simulink model "Simultation"  (R2023b)
settings: Solver=VariableStepAuto  StartTime=0.0  StopTime=25  RelTol=1e-3
values from neighbouring files (symbols this model uses):
  A = M1^(-1)*M2    [QUBE2_Control_System.m]
  B = M1^(-1)*M3    [QUBE2_Control_System.m]
  C = [1,0,0,0 ... (first row only)    [QUBE2_Control_System.m]
  D = 0    [QUBE2_Control_System.m]
  K = [0, 0; 0, g*l1*m1]    [QUBE2_Control_System.m]
undefined symbols (not defined in the file or in its folder): A_swingup, alpha_0, alpha_0_swingup, B_swingup, Bp_, C_swingup, D_swingup, g_, Jp_, Jr_ex_, K_lq, K_swingup, Kc_, Ke_, Lp, lp_, Lr_, mp_, mr, Ra_, theta_0, Va_0
libraries: simulink_extras x36
(part 1 of 2)
settings Model: Creator=mozar  LastModifiedBy=mozar
settings SolverCC: ZeroCrossAlgorithm=Adaptive
settings DebuggingCC: IgnoredZcDiagnostic=none

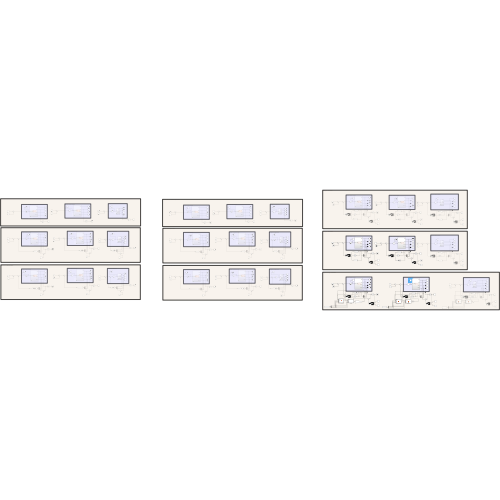
[thumbnail: Simulink's stored preview of the top-level diagram]
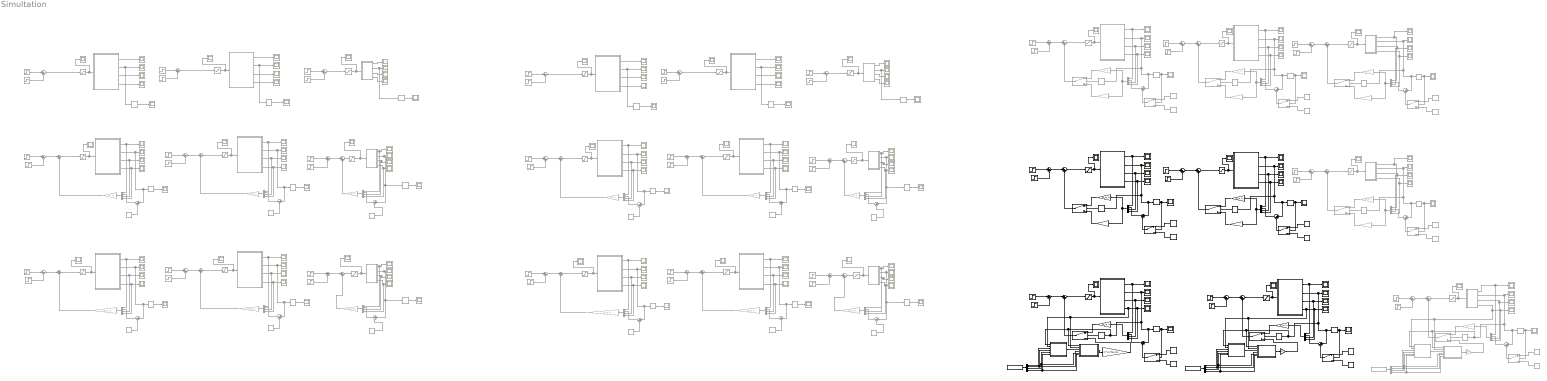
== system Simultation ==
  note: PP Swingup + PP Stabilization
  note: PP - 0 phi - 2V 0.05s Square Disturb
  note: Natual Response - 0 phi - Disturb 2V square 0.05 sec
  note: Complete Linear With Friction
  note: complete nonlinear with friction
  note: complete nonlinear no friction
  note: complete nonlinear no friction
  note: Complete Linear With Friction
  note: complete nonlinear with friction
  note: Complete Linear With Friction
  note: complete nonlinear with friction
  note: complete nonlinear no friction
  note: LQR - 0 phi - 2V 0.05s Square Disturb
  note: Complete Linear With Friction
  note: complete nonlinear with friction
  note: complete nonlinear no friction
  note: complete nonlinear no friction
  note: complete nonlinear with friction
  note: complete nonlinear no friction
  note: LQR - pi phi - 2V 0.05s Square Disturb
  note: Natual Response - pi phi - Disturb 2V square 0.05 sec
  note: complete nonlinear with friction
  note: PP - pi phi - 2V 0.05s Square Disturb
  note: Complete Linear With Friction
  note: Complete Linear With Friction
  note: complete nonlinear no friction
  note: complete nonlinear with friction
  note: Complete Linear With Friction
  note: PP Swingup + LQR Stabilization
  note: complete nonlinear no friction
  note: complete nonlinear with friction
  note: Complete Linear With Friction
  note: Energy Based Swingup + PP Stabilization
  note: complete nonlinear no friction
  note: complete nonlinear with friction
  note: complete linear with friction
  Constant{,1..12,14,17,22,31} (17 alike) : Constant  Commented=on  Value=pi
  Constant{13,18,25,28} (4 alike) : Constant  Value=pi
  Constant{15..16,19,23,32} (5 alike) : Constant  Commented=on  Value=0
  Constant{20..21,27,29} (4 alike) : Constant  Value=0
  Constant24 : Constant  Value=[Jp_ mp_ Lp g_]
  Constant26 : Constant  Value=[Jp_ mp_ Lp g_]
  Constant30 : Constant  Commented=on  Value=[Jp_ mp_ Lp g_]
  Demux1 : Demux
  Demux2 : Demux
  Demux3 : Demux  Commented=on
  Energy computation : MATLAB Function  TreatAsAtomicUnit=on
  Energy computation1 : MATLAB Function  TreatAsAtomicUnit=on
  Energy computation2 : MATLAB Function  Commented=on  TreatAsAtomicUnit=on
  Gain{1..2,6..8,12,19} (7 alike) : Gain  Commented=on  Gain=-K_lq  Multiplication=Matrix(K*u) (u vector)
  Gain{3..5,9..11,13..15,30} (10 alike) : Gain  Commented=on  Gain=-K  Multiplication=Matrix(K*u) (u vector)
  Gain{16..18,24} (4 alike) : Gain  Commented=on  Gain=-K_swingup  Multiplication=Matrix(K*u) (u vector)
  Gain{20..21,27..28} (4 alike) : Gain  Gain=-K_lq  Multiplication=Matrix(K*u) (u vector)
  Gain22 : Gain  Gain=-K_swingup  Multiplication=Matrix(K*u) (u vector)
  Gain23 : Gain  Gain=-K_swingup  Multiplication=Matrix(K*u) (u vector)
  Gain25 : Gain  Gain=mr*Lr_*Ra_/Kc_
  Gain26 : Gain  Gain=mr*Lr_*Ra_/Kc_
  Gain29 : Gain  Commented=on  Gain=mr*Lr_*Ra_/Kc_
  Mux{1..16,20} (17 alike) : Mux  Commented=on
  Mux{17..19,21} (4 alike) : Mux
  Radians to Degrees{,1..23,26,29,34..35} (28 alike) : simulink_extras/Transformations/Radians to Degrees  Commented=on
  Radians to Degrees{24..25,27..28,30..33} (8 alike) : simulink_extras/Transformations/Radians to Degrees
  Saturation{,1..6,9..15,18..20,23,26} (19 alike) : Saturate  Commented=on  UpperLimit=10  LowerLimit=-10
  Saturation{7..8,16..17} (4 alike) : Saturate  Commented=on
  Saturation{21..22,24..25} (4 alike) : Saturate  UpperLimit=10  LowerLimit=-10
  Scope{,1..113,115..126,132..135,142..143,156..161} (138 alike) : Scope  Commented=on
  Scope{114,127..131,136..141,144..155} (24 alike) : Scope
  Step{1,3,5..6,8,10,12,14,16,19..20,22,24,26,30,32..33,35,37,39,41,47,53} (23 alike) : Step  Commented=on  Before=1  After=3  SampleTime=0
  Step{2,4,7,9,11,13,15,17..18,21,23,25,27..29,31,34,36,38,40,42,48,54} (23 alike) : Step  Commented=on  Time=1.05  Before=1  After=3  SampleTime=0
  Step{43,45,49,51} (4 alike) : Step  Before=1  After=3  SampleTime=0
  Step{44,46,50,52} (4 alike) : Step  Time=1.05  Before=1  After=3  SampleTime=0
  Subsystem1 : Subsystem  Commented=on
  Subsystem10 : Subsystem  Commented=on
  Subsystem11 : Subsystem  Commented=on
  Subsystem12 : Subsystem  Commented=on
  Subsystem13 : Subsystem  Commented=on
  Subsystem14 : Subsystem
  Subsystem15 : Subsystem  Commented=on
  Subsystem16 : Subsystem
  Subsystem17 : Subsystem
  Subsystem18 : Subsystem
  Subsystem2 : Subsystem  Commented=on
  Subsystem3 : Subsystem  Commented=on
  Subsystem4 : Subsystem  Commented=on
  Subsystem5 : Subsystem  Commented=on
  Subsystem6 : Subsystem  Commented=on
  Subsystem7 : Subsystem  Commented=on
  Subsystem8 : Subsystem  Commented=on
  Subsystem9 : Subsystem  Commented=on
  Sum{1,5,7,12,16,18,22,25,29,31,38,40,43,46,49,55,67} (17 alike) : Sum  Commented=on  Inputs=|++
  Sum{2..4,6,8..11,13..15,17,19..21,23..24,26..28,30,32..37,39,41..42,44..45,47..48,50..51,56..57,68..69} (40 alike) : Sum  Commented=on  Inputs=|+-
  Sum{52,58,61,64} (4 alike) : Sum  Inputs=|++
  Sum{53..54,59..60,62..63,65..66} (8 alike) : Sum  Inputs=|+-
  Switch{,2,4,10} (4 alike) : Switch  Commented=on  Threshold=135  SaturateOnIntegerOverflow=off  InputSameDT=off
  Switch{1,3,5,11} (4 alike) : Switch  Commented=on  Criteria=u2 > Threshold  Threshold=135  SaturateOnIntegerOverflow=off  InputSameDT=off
  Switch12 : Switch  Threshold=155  SaturateOnIntegerOverflow=off  InputSameDT=off
  Switch13 : Switch  Criteria=u2 > Threshold  Threshold=155  SaturateOnIntegerOverflow=off  InputSameDT=off
  Switch{6,8,14..15} (4 alike) : Switch  Threshold=135  SaturateOnIntegerOverflow=off  InputSameDT=off
  Switch16 : Switch  Commented=on  Threshold=155  SaturateOnIntegerOverflow=off  InputSameDT=off
  Switch17 : Switch  Commented=on  Criteria=u2 > Threshold  Threshold=155  SaturateOnIntegerOverflow=off  InputSameDT=off
  Switch7 : Switch  Criteria=u2 > Threshold  Threshold=135  SaturateOnIntegerOverflow=off  InputSameDT=off
  Switch9 : Switch  Criteria=u2 > Threshold  Threshold=135  SaturateOnIntegerOverflow=off  InputSameDT=off
  linearized_model1 : Subsystem  Commented=on
  linearized_model2 : Subsystem  Commented=on
  linearized_model3 : Subsystem  Commented=on
  linearized_model4 : Subsystem  Commented=on
  linearized_model5 : Subsystem  Commented=on
  linearized_model6 : Subsystem  Commented=on
  linearized_model7 : Subsystem  Commented=on
  linearized_model8 : Subsystem  Commented=on
  linearized_model9 : Subsystem  Commented=on
  saturation : MATLAB Function  TreatAsAtomicUnit=on
  saturation1 : MATLAB Function  TreatAsAtomicUnit=on
  saturation2 : MATLAB Function  Commented=on  TreatAsAtomicUnit=on
  wires:
  linearized_model1/2(alpha) -> Radians to Degrees3/1, Scope19/1
  linearized_model1/1(theta) -> Scope18/1
  Radians to Degrees3/1 -> Scope20/1
  linearized_model1/4(alpha_d) -> Scope17/1
  linearized_model1/3(theta_d) -> Scope16/1
  Subsystem2/1(theta) -> Scope21/1
  Subsystem2/4(alpha_d) -> Scope24/1
  Sum10/1 -> Saturation2/1
  Subsystem2/2(alpha) -> Radians to Degrees4/1, Scope22/1
  Saturation2/1 -> Scope50/1, Subsystem2/1(Input_Voltage)
  Subsystem2/3(theta_d) -> Scope23/1
  Radians to Degrees4/1 -> Scope25/1
  Saturation3/1 -> Scope31/1, Subsystem3/1(Input_Voltage)
  Subsystem3/2(alpha) -> Radians to Degrees5/1, Scope27/1
  Subsystem3/3(theta_d) -> Scope28/1
  Step11/1 -> Sum9/2
  Radians to Degrees5/1 -> Scope30/1
  Step10/1 -> Sum9/1
  Subsystem3/4(alpha_d) -> Scope29/1
  Sum9/1 -> Saturation3/1
  Subsystem3/1(theta) -> Scope26/1
  Step6/1 -> Sum10/1
  Step7/1 -> Sum10/2
  Step8/1 -> Sum11/1
  Step9/1 -> Sum11/2
  Subsystem4/1(theta) -> Mux3/1, Scope32/1
  Mux3/1 -> Gain3/1
  Radians to Degrees6/1 -> Scope36/1
  Constant3/1 -> Sum14/2
  Subsystem4/4(alpha_d) -> Mux3/4, Scope35/1
  Sum12/1 -> Saturation4/1
  Subsystem4/2(alpha) -> Sum14/1, Radians to Degrees6/1, Scope33/1
  Sum14/1 -> Mux3/2
  Sum13/1 -> Sum12/1
  Saturation4/1 -> Scope/1, Subsystem4/1(Input_Voltage)
  Subsystem4/3(theta_d) -> Mux3/3, Scope34/1
  Gain3/1 -> Sum12/2
  linearized_model2/2(alpha) -> Sum15/1, Radians to Degrees7/1, Scope40/1
  Mux4/1 -> Gain4/1
  linearized_model2/1(theta) -> Mux4/1, Scope39/1
  Radians to Degrees7/1 -> Scope41/1
  Gain4/1 -> Sum16/2
  Sum17/1 -> Sum16/1
  Constant4/1 -> Sum15/2
  linearized_model2/4(alpha_d) -> Mux4/4, Scope38/1
  Sum15/1 -> Mux4/2
  linearized_model2/3(theta_d) -> Mux4/3, Scope37/1
  Subsystem5/2(alpha) -> Sum20/1, Radians to Degrees8/1, Scope43/1
  Saturation5/1 -> Scope42/1, Subsystem5/1(Input_Voltage)
  Sum19/1 -> Sum18/1
  Subsystem5/3(theta_d) -> Mux5/3, Scope44/1
  Subsystem5/4(alpha_d) -> Mux5/4, Scope45/1
  Radians to Degrees8/1 -> Scope46/1
  Subsystem5/1(theta) -> Mux5/1, Scope47/1
  Mux5/1 -> Gain5/1
  Sum18/1 -> Saturation5/1
  Constant5/1 -> Sum20/2
  Gain5/1 -> Sum18/2
  Sum20/1 -> Mux5/2
  Step12/1 -> Sum13/1
  Step13/1 -> Sum13/2
  Step14/1 -> Sum19/1
  Step15/1 -> Sum19/2
  Step16/1 -> Sum17/1
  Step17/1 -> Sum17/2
  Sum6/1 -> Sum5/1
  Sum4/1 -> Mux2/2
  Constant2/1 -> Sum4/2
  linearized_model3/4(alpha_d) -> Mux2/4, Scope7/1
  linearized_model3/3(theta_d) -> Mux2/3, Scope6/1
  Mux2/1 -> Gain2/1
  linearized_model3/1(theta) -> Mux2/1, Scope8/1
  Sum7/1 -> Saturation6/1
  Mux6/1 -> Gain6/1
  Radians to Degrees2/1 -> Scope10/1
  Sum21/1 -> Mux6/2
  Subsystem6/1(theta) -> Mux6/1, Scope15/1
  Saturation6/1 -> Scope52/1, Subsystem6/1(Input_Voltage)
  linearized_model3/2(alpha) -> Sum4/1, Radians to Degrees2/1, Scope9/1
  Subsystem6/3(theta_d) -> Mux6/3, Scope12/1
  Step5/1 -> Sum6/1
  Radians to Degrees9/1 -> Scope14/1
  Sum8/1 -> Sum7/1
  Step3/1 -> Sum8/1
  Constant6/1 -> Sum21/2
  Step1/1 -> Sum2/1
  Step2/1 -> Sum2/2
  Subsystem6/2(alpha) -> Sum21/1, Radians to Degrees9/1, Scope11/1
  Step4/1 -> Sum8/2
  Sum2/1 -> Sum1/1
  Saturation1/1 -> Scope51/1, Subsystem1/1(Input_Voltage)
  Gain6/1 -> Sum7/2
  Gain1/1 -> Sum1/2
  Gain2/1 -> Sum5/2
  Subsystem1/3(theta_d) -> Mux1/3, Scope3/1
  Constant1/1 -> Sum3/2
  Subsystem1/1(theta) -> Mux1/1, Scope1/1
  Mux1/1 -> Gain1/1
  Subsystem6/4(alpha_d) -> Mux6/4, Scope13/1
  Radians to Degrees1/1 -> Scope5/1
  Sum1/1 -> Saturation1/1
  Step18/1 -> Sum6/2
  Subsystem1/2(alpha) -> Sum3/1, Radians to Degrees1/1, Scope2/1
  Sum3/1 -> Mux1/2
  Subsystem1/4(alpha_d) -> Mux1/4, Scope4/1
  Sum16/1 -> Saturation/1
  Saturation/1 -> Scope48/1, linearized_model2/1(Va)
  Saturation7/1 -> Scope49/1, linearized_model1/1(Va)
  Sum11/1 -> Saturation7/1
  Sum5/1 -> Saturation8/1
  Saturation8/1 -> Scope53/1, linearized_model3/1(Va)
  Sum30/1 -> Sum29/1
  Sum28/1 -> Mux10/2
  Constant10/1 -> Sum28/2
  linearized_model5/4(alpha_d) -> Mux10/4, Scope86/1
  Step26/1 -> Sum30/1
  Gain10/1 -> Sum29/2
  Mux10/1 -> Gain10/1
  linearized_model5/1(theta) -> Mux10/1, Scope87/1
  linearized_model5/2(alpha) -> Sum28/1, Radians to Degrees16/1, Scope89/1
  Sum31/1 -> Saturation14/1
  Gain11/1 -> Sum31/2
  Mux11/1 -> Gain11/1
  Sum34/1 -> Mux11/2
  Subsystem11/1(theta) -> Mux11/1, Scope96/1
  Saturation14/1 -> Scope91/1, Subsystem11/1(Input_Voltage)
  Radians to Degrees17/1 -> Scope95/1
  Sum32/1 -> Sum31/1
  Subsystem11/4(alpha_d) -> Mux11/4, Scope94/1
  Subsystem11/2(alpha) -> Sum34/1, Radians to Degrees17/1, Scope92/1
  Step24/1 -> Sum32/1
  Step22/1 -> Sum26/1
  Step23/1 -> Sum26/2
  Step25/1 -> Sum32/2
  Sum26/1 -> Sum25/1
  Saturation13/1 -> Scope54/1, Subsystem10/1(Input_Voltage)
  Subsystem10/3(theta_d) -> Mux9/3, Scope82/1
  Subsystem10/1(theta) -> Mux9/1, Scope80/1
  Mux9/1 -> Gain9/1
  Sum25/1 -> Saturation13/1
  Step35/1 -> Sum24/1
  Saturation11/1 -> Scope100/1, Subsystem8/1(Input_Voltage)
  Subsystem11/3(theta_d) -> Mux11/3, Scope93/1
  Subsystem8/2(alpha) -> Radians to Degrees13/1, Scope69/1
  Subsystem8/1(theta) -> Scope68/1
  Subsystem8/3(theta_d) -> Scope70/1
  Subsystem8/4(alpha_d) -> Scope71/1
  Step36/1 -> Sum24/2
  Radians to Degrees13/1 -> Scope72/1
  Sum23/1 -> Saturation11/1
  Sum27/1 -> Mux9/2
  Step20/1 -> Sum42/1
  Step21/1 -> Sum42/2
  Constant11/1 -> Sum34/2
  Sum42/1 -> Saturation12/1
  Radians to Degrees14/1 -> Scope78/1
  Sum38/1 -> Saturation17/1
  Gain9/1 -> Sum25/2
  Saturation17/1 -> Scope103/1, linearized_model6/1(Va)
  Step27/1 -> Sum30/2
  Sum29/1 -> Saturation9/1
  Sum24/1 -> Saturation16/1
  Saturation16/1 -> Scope98/1, linearized_model4/1(Va)
  Step34/1 -> Sum23/2
  Subsystem9/1(theta) -> Scope73/1
  Subsystem9/3(theta_d) -> Scope75/1
  Constant9/1 -> Sum27/2
  Subsystem9/4(alpha_d) -> Scope76/1
  Subsystem7/4(alpha_d) -> Mux7/4, Scope88/1
  Subsystem12/4(alpha_d) -> Mux12/4, Scope59/1
  Radians to Degrees10/1 -> Scope99/1
  Mux7/1 -> Gain7/1
  Sum36/1 -> Mux7/2
  Step28/1 -> Sum39/2
  Subsystem7/3(theta_d) -> Mux7/3, Scope77/1
  Subsystem7/2(alpha) -> Sum36/1, Radians to Degrees10/1, Scope66/1
  Subsystem12/2(alpha) -> Sum35/1, Radians to Degrees18/1, Scope57/1
  Radians to Degrees15/1 -> Scope84/1
  Step29/1 -> Sum33/2
  Step31/1 -> Sum41/2
  Radians to Degrees16/1 -> Scope90/1
  Gain12/1 -> Sum40/2
  Sum33/1 -> Sum22/1
  Subsystem12/3(theta_d) -> Mux12/3, Scope58/1
  Sum41/1 -> Sum40/1
  Radians to Degrees18/1 -> Scope60/1
  Gain8/1 -> Sum38/2
  Constant12/1 -> Sum35/2
  Radians to Degrees11/1 -> Scope56/1
  Subsystem10/4(alpha_d) -> Mux9/4, Scope83/1
  Subsystem9/2(alpha) -> Radians to Degrees14/1, Scope74/1
  Sum40/1 -> Saturation15/1
  Saturation10/1 -> Scope101/1, Subsystem7/1(Input_Voltage)
  Constant7/1 -> Sum36/2
  Mux12/1 -> Gain12/1
  Subsystem12/1(theta) -> Mux12/1, Scope61/1
  Step30/1 -> Sum41/1
  Step19/1 -> Sum33/1
  linearized_model6/3(theta_d) -> Mux8/3, Scope104/1
  linearized_model6/4(alpha_d) -> Mux8/4, Scope105/1
  linearized_model6/2(alpha) -> Sum37/1, Radians to Degrees11/1, Scope107/1
  Gain7/1 -> Sum22/2
  linearized_model5/3(theta_d) -> Mux10/3, Scope85/1
  Step33/1 -> Sum23/1
  Step32/1 -> Sum39/1
  Sum39/1 -> Sum38/1
  Sum37/1 -> Mux8/2
  Subsystem7/1(theta) -> Mux7/1, Scope55/1
  Mux8/1 -> Gain8/1
  Sum22/1 -> Saturation10/1
  linearized_model6/1(theta) -> Mux8/1, Scope106/1
  Saturation12/1 -> Scope79/1, Subsystem9/1(Input_Voltage)
  linearized_model4/1(theta) -> Scope64/1
  Sum35/1 -> Mux12/2
  Saturation9/1 -> Scope97/1, linearized_model5/1(Va)
  Radians to Degrees12/1 -> Scope67/1
  linearized_model4/3(theta_d) -> Scope62/1
  Constant8/1 -> Sum37/2
  Subsystem10/2(alpha) -> Sum27/1, Radians to Degrees15/1, Scope81/1
  linearized_model4/2(alpha) -> Radians to Degrees12/1, Scope65/1
  linearized_model4/4(alpha_d) -> Scope63/1
  Saturation15/1 -> Scope102/1, Subsystem12/1(Input_Voltage)
  Step38/1 -> Sum44/2
  Radians to Degrees19/1 -> Scope113/1, Switch1/2
  Sum45/1 -> Mux15/2
  Sum43/1 -> Saturation18/1
  Saturation18/1 -> Subsystem13/1(Input_Voltage), Scope108/1
  Subsystem13/1(theta) -> Mux15/1, Scope109/1
  Subsystem13/3(theta_d) -> Mux15/3, Scope111/1
  Step37/1 -> Sum44/1
  Sum44/1 -> Sum43/1
  Subsystem13/4(alpha_d) -> Mux15/4, Scope112/1
  Subsystem13/2(alpha) -> Radians to Degrees/1, Sum45/1, Radians to Degrees19/1, Scope110/1
  Switch/1 -> Sum43/2
  Mux15/1 -> Gain16/1, Gain15/1
  Gain16/1 -> Switch/3
  Gain15/1 -> Switch/1
  Radians to Degrees/1 -> Switch/2
  Switch1/1 -> Sum45/2
  Constant/1 -> Switch1/1
  Constant15/1 -> Switch1/3
  Radians to Degrees21/1 -> Switch2/2
  Mux14/1 -> Gain17/1, Gain14/1
  Gain17/1 -> Switch2/3
  Gain14/1 -> Switch2/1
  Subsystem15/4(alpha_d) -> Mux14/4, Scope123/1
  Switch3/1 -> Sum51/2
  Subsystem15/3(theta_d) -> Mux14/3, Scope122/1
  Sum50/1 -> Sum49/1
  Subsystem15/2(alpha) -> Radians to Degrees21/1, Sum51/1, Radians to Degrees22/1, Scope121/1
  Step39/1 -> Sum50/1
  Subsystem15/1(theta) -> Mux14/1, Scope120/1
  Saturation19/1 -> Subsystem15/1(Input_Voltage), Scope119/1
  Sum49/1 -> Saturation19/1
  Radians to Degrees22/1 -> Scope124/1, Switch3/2
  Switch2/1 -> Sum49/2
  Constant14/1 -> Switch3/1
  Step40/1 -> Sum50/2
  Constant16/1 -> Switch3/3
  Sum51/1 -> Mux14/2
  linearized_model8/3(theta_d) -> Mux13/3, Scope118/1
  linearized_model8/2(alpha) -> Scope117/1, Radians to Degrees20/1, Sum48/1, Radians to Degrees23/1
  linearized_model8/1(theta) -> Scope116/1, Mux13/1
  Saturation20/1 -> linearized_model8/1(Va), Scope115/1
  Step42/1 -> Sum47/2
  Constant19/1 -> Switch5/3
  Switch4/1 -> Sum46/2
  Radians to Degrees23/1 -> Scope126/1, Switch5/2
  Sum46/1 -> Saturation20/1
  Sum47/1 -> Sum46/1
  Switch5/1 -> Sum48/2
  Step41/1 -> Sum47/1
  Sum48/1 -> Mux13/2
  Radians to Degrees20/1 -> Switch4/2
  Mux13/1 -> Gain18/1, Gain13/1
  Gain13/1 -> Switch4/1
  Gain18/1 -> Switch4/3
  linearized_model8/4(alpha_d) -> Mux13/4, Scope125/1
  Constant17/1 -> Switch5/1
  Constant22/1 -> Switch11/1
  Radians to Degrees28/1 -> Scope141/1, Switch9/2
  Sum59/1 -> Sum58/1
  Subsystem16/1(theta) -> Mux17/1, Scope137/1
  linearized_model7/1(theta) -> Scope133/1, Mux16/1
  Radians to Degrees29/1 -> Scope143/1, Switch11/2
  Constant18/1 -> Switch9/1
  Sum60/1 -> Mux17/2
  Constant20/1 -> Switch7/3
  Step44/1 -> Sum53/2
  Step46/1 -> Sum59/2
  Switch8/1 -> Sum58/2
  Step43/1 -> Sum53/1
  Sum52/1 -> Saturation21/1
  Radians to Degrees25/1 -> Scope131/1, Switch7/2
  Subsystem16/4(alpha_d) -> Mux17/4, Scope140/1
  Switch9/1 -> Sum60/2
  Gain20/1 -> Switch8/1
  Constant13/1 -> Switch7/1
  Gain22/1 -> Switch6/3
  Switch6/1 -> Sum52/2
  Sum58/1 -> Saturation22/1
  Mux16/1 -> Gain24/1, Gain19/1
  Step48/1 -> Sum56/2
  linearized_model7/2(alpha) -> Scope134/1, Radians to Degrees26/1, Sum57/1, Radians to Degrees29/1
  Radians to Degrees27/1 -> Switch8/2
  Gain19/1 -> Switch10/1
  Subsystem16/3(theta_d) -> Mux17/3, Scope139/1
  Sum53/1 -> Sum52/1
  Mux17/1 -> Gain23/1, Gain20/1
  Radians to Degrees26/1 -> Switch10/2
  Constant21/1 -> Switch9/3
  Subsystem16/2(alpha) -> Radians to Degrees27/1, Sum60/1, Radians to Degrees28/1, Scope138/1
  Sum57/1 -> Mux16/2
  linearized_model7/3(theta_d) -> Mux16/3, Scope135/1
  Step47/1 -> Sum56/1
  Saturation21/1 -> Subsystem14/1(Input_Voltage), Scope114/1
  Saturation22/1 -> Subsystem16/1(Input_Voltage), Scope136/1
  Gain21/1 -> Switch6/1
  Constant23/1 -> Switch11/3
  Switch10/1 -> Sum55/2
  Switch7/1 -> Sum54/2
  Sum56/1 -> Sum55/1
  Sum55/1 -> Saturation23/1
  Sum54/1 -> Mux18/2
  Saturation23/1 -> linearized_model7/1(Va), Scope132/1
  Switch11/1 -> Sum57/2
  Radians to Degrees24/1 -> Switch6/2
  Step45/1 -> Sum59/1
  Gain24/1 -> Switch10/3
  linearized_model7/4(alpha_d) -> Mux16/4, Scope142/1
  Subsystem14/1(theta) -> Mux18/1, Scope127/1
  Subsystem14/4(alpha_d) -> Mux18/4, Scope130/1
  Gain23/1 -> Switch8/3
  Subsystem14/2(alpha) -> Radians to Degrees24/1, Sum54/1, Radians to Degrees25/1, Scope128/1
  Subsystem14/3(theta_d) -> Mux18/3, Scope129/1
  Mux18/1 -> Gain22/1, Gain21/1
  Demux2/4 -> Energy computation/6(g0), saturation/6(g0)
  saturation/1(u) -> Gain25/1
  Constant24/1 -> Demux2/1
  Demux2/1 -> Energy computation/3(Ip)
  Energy computation/1(E) -> saturation/3(E)
  Demux2/2 -> saturation/4(mp), Energy computation/4(mp)
  Demux2/3 -> saturation/5(Lp), Energy computation/5(Lp)
  Radians to Degrees31/1 -> Scope149/1, Switch15/2
  Constant27/1 -> Switch15/3
  Step50/1 -> Sum62/2
  Subsystem17/2(alpha) -> saturation/1(phi), Energy computation/1(phi), Radians to Degrees30/1, Sum63/1, Radians to Degrees31/1, Scope146/1
  Subsystem17/3(theta_d) -> Mux21/3, Scope147/1
  Mux21/1 -> Gain28/1
  Subsystem17/1(theta) -> Mux21/1, Scope145/1
  Radians to Degrees30/1 -> Switch14/2
  Sum63/1 -> Mux21/2
  Step49/1 -> Sum62/1
  Sum61/1 -> Saturation24/1
  Saturation24/1 -> Subsystem17/1(Input_Voltage), Scope144/1
  Subsystem17/4(alpha_d) -> saturation/2(phi_dot), Energy computation/2(phi_dot), Mux21/4, Scope148/1
  Sum62/1 -> Sum61/1
  Switch14/1 -> Sum61/2
  Constant25/1 -> Switch15/1
  Switch15/1 -> Sum63/2
  Gain28/1 -> Switch14/1
  Gain25/1 -> Switch14/3
  saturation1/1(u) -> Gain26/1
  Gain27/1 -> Switch12/1
  Constant26/1 -> Demux1/1
  Sum65/1 -> Sum64/1
  Saturation25/1 -> Subsystem18/1(Input_Voltage), Scope150/1
  Switch13/1 -> Sum66/2
  Constant28/1 -> Switch13/1
  Demux1/3 -> saturation1/5(Lp), Energy computation1/5(Lp)
  Demux1/2 -> saturation1/4(mp), Energy computation1/4(mp)
  Demux1/4 -> Energy computation1/6(g0), saturation1/6(g0)
  Demux1/1 -> Energy computation1/3(Ip)
  Switch12/1 -> Sum64/2
  Sum66/1 -> Mux19/2
  Subsystem18/4(alpha_d) -> Mux19/4, Scope154/1, saturation1/2(phi_dot), Energy computation1/2(phi_dot)
  Radians to Degrees33/1 -> Scope155/1, Switch13/2
  Mux19/1 -> Gain27/1
  Gain26/1 -> Switch12/3
  Subsystem18/1(theta) -> Mux19/1, Scope151/1
  Subsystem18/2(alpha) -> saturation1/1(phi), Energy computation1/1(phi), Radians to Degrees32/1, Sum66/1, Radians to Degrees33/1, Scope152/1
  Sum64/1 -> Saturation25/1
  Constant29/1 -> Switch13/3
  Subsystem18/3(theta_d) -> Mux19/3, Scope153/1
  Energy computation1/1(E) -> saturation1/3(E)
  Radians to Degrees32/1 -> Switch12/2
  Step51/1 -> Sum65/1
  Step52/1 -> Sum65/2
  saturation2/1(u) -> Gain29/1
  Gain30/1 -> Switch16/1
  Constant30/1 -> Demux3/1
  Sum68/1 -> Sum67/1
  Saturation26/1 -> linearized_model9/1(Va), Scope156/1
  Switch17/1 -> Sum69/2
  Constant31/1 -> Switch17/1
  Demux3/3 -> saturation2/5(Lp), Energy computation2/5(Lp)
  Demux3/2 -> saturation2/4(mp), Energy computation2/4(mp)
  Demux3/4 -> Energy computation2/6(g0), saturation2/6(g0)
  Demux3/1 -> Energy computation2/3(Ip)
  Switch16/1 -> Sum67/2
  Sum69/1 -> Mux20/2
  linearized_model9/4(alpha_d) -> saturation2/2(phi_dot), Energy computation2/2(phi_dot), Mux20/4, Scope160/1
  Radians to Degrees35/1 -> Scope161/1, Switch17/2
  Mux20/1 -> Gain30/1
  Gain29/1 -> Switch16/3
  linearized_model9/1(theta) -> Mux20/1, Scope157/1
  linearized_model9/2(alpha) -> Scope158/1, saturation2/1(phi), Energy computation2/1(phi), Radians to Degrees34/1, Sum69/1, Radians to Degrees35/1
  Sum67/1 -> Saturation26/1
  Constant32/1 -> Switch17/3
  linearized_model9/3(theta_d) -> Mux20/3, Scope159/1
  Energy computation2/1(E) -> saturation2/3(E)
  Radians to Degrees34/1 -> Switch16/2
  Step53/1 -> Sum68/1
  Step54/1 -> Sum68/2

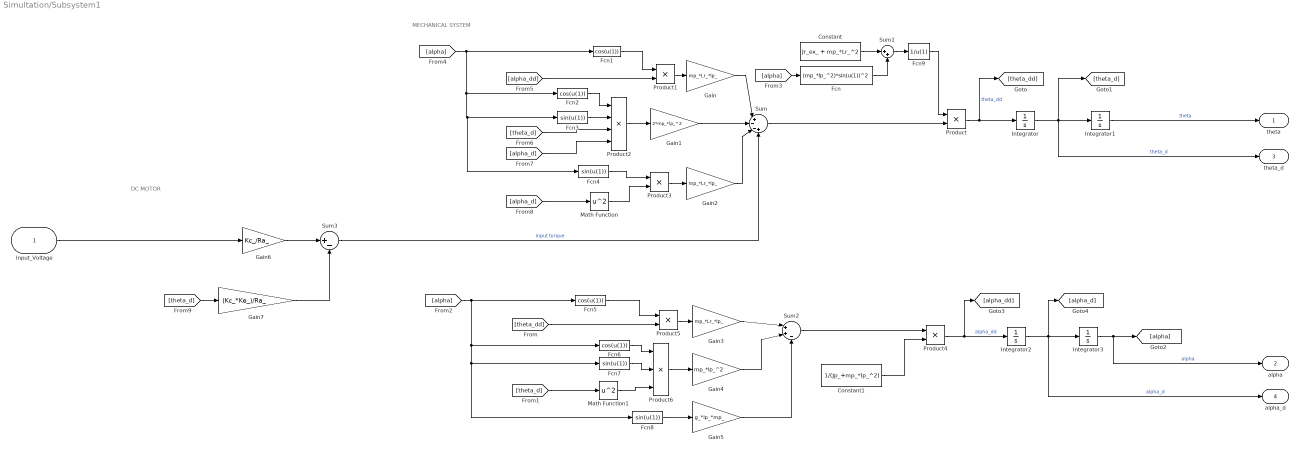
== system Simultation/Subsystem1 ==
  note: DC MOTOR
  note: MECHANICAL SYSTEM
  Input_Voltage : Inport
  Constant : Constant  Value=Jr_ex_ + mp_*Lr_^2
  Constant1 : Constant  Value=1/(Jp_+mp_*lp_^2)
  Fcn : Fcn  Expr=(mp_*lp_^2)*sin(u(1))^2
  Fcn{1..2,5..6} (4 alike) : Fcn  Expr=cos(u(1))
  Fcn{3..4,7..8} (4 alike) : Fcn  Expr=sin(u(1))
  Fcn9 : Fcn  Expr=1/u(1)
  Gain : Gain  Gain=mp_*Lr_*lp_
  Gain1 : Gain  Gain=2*mp_*lp_^2
  Gain2 : Gain  Gain=mp_*Lr_*lp_
  Gain3 : Gain  Gain=mp_*Lr_*lp_
  Gain4 : Gain  Gain=mp_*lp_^2
  Gain5 : Gain  Gain=g_*lp_*mp_
  Gain6 : Gain  Gain=Kc_/Ra_
  Gain7 : Gain  Gain=(Kc_*Ke_)/Ra_
  Integrator{,1..3} (4 alike) : Integrator
  Math Function : Math  Operator=square
  Math Function1 : Math  Operator=square
  Product{,1,3..5} (5 alike) : Product
  Product2 : Product  Inputs=4
  Product6 : Product  Inputs=3
  Sum : Sum  Inputs=|+--+
  Sum1 : Sum  Inputs=|++
  Sum2 : Sum  Inputs=|++-
  Sum3 : Sum  Inputs=|+-
  theta : Outport
  alpha : Outport  Port=2
  theta_d : Outport  Port=3
  alpha_d : Outport  Port=4
  wires:
  Integrator2/1 -> alpha_d/1, Integrator3/1, [alpha_d]  "alpha_d"
  Fcn6/1 -> Product6/1
  Product4/1 -> [alpha_dd], Integrator2/1  "alpha_dd"
  Fcn4/1 -> Product3/1
  Integrator/1 -> theta_d/1, [theta_d], Integrator1/1  "theta_d"
  Gain1/1 -> Sum/2
  Gain6/1 -> Sum3/1
  Fcn3/1 -> Product2/2
  Fcn1/1 -> Product1/1
  Integrator1/1 -> theta/1  "theta"
  Fcn8/1 -> Gain5/1
  Fcn7/1 -> Product6/2
  Gain5/1 -> Sum2/3
  Sum1/1 -> Fcn9/1
  Fcn/1 -> Sum1/2
  Product1/1 -> Gain/1
  Fcn9/1 -> Product/1
  Product3/1 -> Gain2/1
  Sum/1 -> Product/2
  [alpha_d] -> Math Function/1
  [theta_dd] -> Product5/2
  [theta_d] -> Gain7/1
  Product5/1 -> Gain3/1
  Integrator3/1 -> alpha/1, [alpha]  "alpha"
  Fcn5/1 -> Product5/1
  Product6/1 -> Gain4/1
  Sum2/1 -> Product4/1
  Math Function1/1 -> Product6/3
  Math Function/1 -> Product3/2
  Product/1 -> Integrator/1, [theta_dd]  "theta_dd"
  Gain4/1 -> Sum2/2
  Input_Voltage/1 -> Gain6/1
  Constant/1 -> Sum1/1
  [alpha] -> Fcn8/1, Fcn7/1, Fcn6/1, Fcn5/1
  Constant1/1 -> Product4/2
  Product2/1 -> Gain1/1
  [alpha] -> Fcn4/1, Fcn3/1, Fcn2/1, Fcn1/1
  [alpha_d] -> Product2/4
  [alpha_dd] -> Product1/2
  [alpha] -> Fcn/1
  Fcn2/1 -> Product2/1
  Sum3/1 -> Sum/4  "input torque"
  Gain2/1 -> Sum/3
  Gain/1 -> Sum/1
  Gain3/1 -> Sum2/1
  [theta_d] -> Math Function1/1
  Gain7/1 -> Sum3/2
  [theta_d] -> Product2/3

== system Simultation/Subsystem10 ==
  note: DC MOTOR
  note: MECHANICAL SYSTEM
  Input_Voltage : Inport
  Constant : Constant  Value=Jr_ex_ + mp_*Lr_^2
  Constant1 : Constant  Value=1/(Jp_+mp_*lp_^2)
  Fcn : Fcn  Expr=(mp_*lp_^2)*sin(u(1))^2
  Fcn{1..2,5..6} (4 alike) : Fcn  Expr=cos(u(1))
  Fcn{3..4,7..8} (4 alike) : Fcn  Expr=sin(u(1))
  Fcn9 : Fcn  Expr=1/u(1)
  Gain : Gain  Gain=mp_*Lr_*lp_
  Gain1 : Gain  Gain=2*mp_*lp_^2
  Gain2 : Gain  Gain=mp_*Lr_*lp_
  Gain3 : Gain  Gain=mp_*Lr_*lp_
  Gain4 : Gain  Gain=mp_*lp_^2
  Gain5 : Gain  Gain=g_*lp_*mp_
  Gain6 : Gain  Gain=Kc_/Ra_
  Gain7 : Gain  Gain=(Kc_*Ke_)/Ra_
  Integrator : Integrator
  Integrator1 : Integrator
  Integrator2 : Integrator
  Integrator3 : Integrator  InitialCondition=pi
  Math Function : Math  Operator=square
  Math Function1 : Math  Operator=square
  Product{,1,3..5} (5 alike) : Product
  Product2 : Product  Inputs=4
  Product6 : Product  Inputs=3
  Sum : Sum  Inputs=|+--+
  Sum1 : Sum  Inputs=|++
  Sum2 : Sum  Inputs=|++-
  Sum3 : Sum  Inputs=|+-
  theta : Outport
  alpha : Outport  Port=2
  theta_d : Outport  Port=3
  alpha_d : Outport  Port=4
  wires:
  Integrator2/1 -> alpha_d/1, Integrator3/1, [alpha_d]  "alpha_d"
  Fcn6/1 -> Product6/1
  Product4/1 -> [alpha_dd], Integrator2/1  "alpha_dd"
  Fcn4/1 -> Product3/1
  Integrator/1 -> theta_d/1, [theta_d], Integrator1/1  "theta_d"
  Gain1/1 -> Sum/2
  Gain6/1 -> Sum3/1
  Fcn3/1 -> Product2/2
  Fcn1/1 -> Product1/1
  Integrator1/1 -> theta/1  "theta"
  Fcn8/1 -> Gain5/1
  Fcn7/1 -> Product6/2
  Gain5/1 -> Sum2/3
  Sum1/1 -> Fcn9/1
  Fcn/1 -> Sum1/2
  Product1/1 -> Gain/1
  Fcn9/1 -> Product/1
  Product3/1 -> Gain2/1
  Sum/1 -> Product/2
  [alpha_d] -> Math Function/1
  [theta_dd] -> Product5/2
  [theta_d] -> Gain7/1
  Product5/1 -> Gain3/1
  Integrator3/1 -> alpha/1, [alpha]  "alpha"
  Fcn5/1 -> Product5/1
  Product6/1 -> Gain4/1
  Sum2/1 -> Product4/1
  Math Function1/1 -> Product6/3
  Math Function/1 -> Product3/2
  Product/1 -> Integrator/1, [theta_dd]  "theta_dd"
  Gain4/1 -> Sum2/2
  Input_Voltage/1 -> Gain6/1
  Constant/1 -> Sum1/1
  [alpha] -> Fcn8/1, Fcn7/1, Fcn6/1, Fcn5/1
  Constant1/1 -> Product4/2
  Product2/1 -> Gain1/1
  [alpha] -> Fcn4/1, Fcn3/1, Fcn2/1, Fcn1/1
  [alpha_d] -> Product2/4
  [alpha_dd] -> Product1/2
  [alpha] -> Fcn/1
  Fcn2/1 -> Product2/1
  Sum3/1 -> Sum/4  "input torque"
  Gain2/1 -> Sum/3
  Gain/1 -> Sum/1
  Gain3/1 -> Sum2/1
  [theta_d] -> Math Function1/1
  Gain7/1 -> Sum3/2
  [theta_d] -> Product2/3

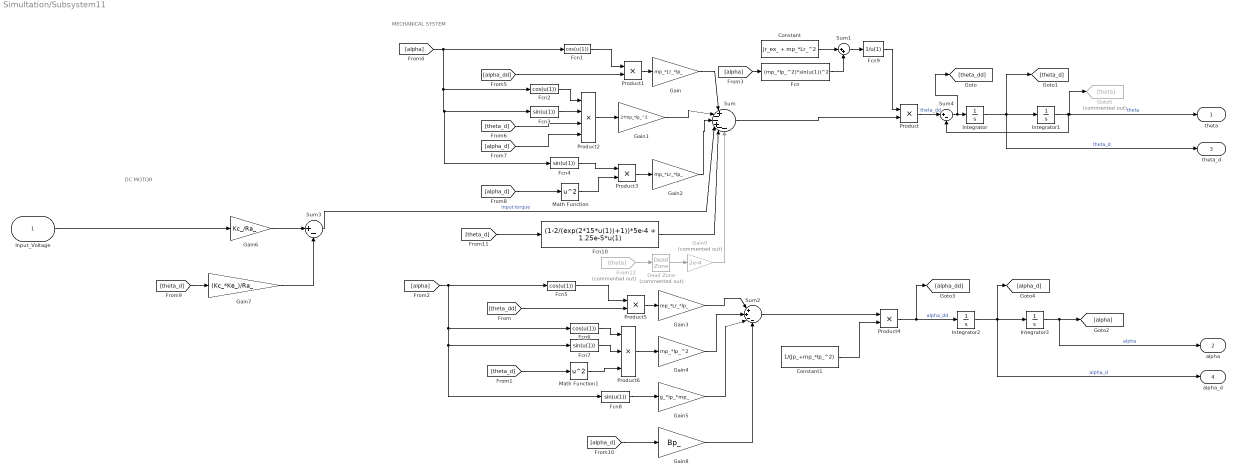
== system Simultation/Subsystem11 ==
  note: MECHANICAL SYSTEM
  note: DC MOTOR
  Input_Voltage : Inport
  Constant : Constant  Value=Jr_ex_ + mp_*Lr_^2
  Constant1 : Constant  Value=1/(Jp_+mp_*lp_^2)
  Dead Zone : DeadZone  Commented=on  LowerValue=0  UpperValue=0  ZeroCross=off
  Fcn : Fcn  Expr=(mp_*lp_^2)*sin(u(1))^2
  Fcn{1..2,5..6} (4 alike) : Fcn  Expr=cos(u(1))
  Fcn10 : Fcn  Expr=(1-2/(exp(2*15*u(1))+1))*5e-4 + 1.25e-5*u(1)
  Fcn{3..4,7..8} (4 alike) : Fcn  Expr=sin(u(1))
  Fcn9 : Fcn  Expr=1/u(1)
  From12 : From  Commented=on  GotoTag=theta
  Gain : Gain  Gain=mp_*Lr_*lp_
  Gain1 : Gain  Gain=2*mp_*lp_^2
  Gain2 : Gain  Gain=mp_*Lr_*lp_
  Gain3 : Gain  Gain=mp_*Lr_*lp_
  Gain4 : Gain  Gain=mp_*lp_^2
  Gain5 : Gain  Gain=g_*lp_*mp_
  Gain6 : Gain  Gain=Kc_/Ra_
  Gain7 : Gain  Gain=(Kc_*Ke_)/Ra_
  Gain8 : Gain  Gain=Bp_
  Gain9 : Gain  Commented=on  Gain=2e-4
  Goto5 : Goto  Commented=on  GotoTag=theta
  Integrator : Integrator
  Integrator1 : Integrator
  Integrator2 : Integrator
  Integrator3 : Integrator  InitialCondition=pi
  Math Function : Math  Operator=square
  Math Function1 : Math  Operator=square
  Product{,1,3..5} (5 alike) : Product
  Product2 : Product  Inputs=4
  Product6 : Product  Inputs=3
  Sum : Sum  Inputs=|+--+--
  Sum1 : Sum  Inputs=|++
  Sum2 : Sum  Inputs=|++--
  Sum3 : Sum  Inputs=|+-
  Sum4 : Sum  Inputs=|+-
  theta : Outport
  alpha : Outport  Port=2
  theta_d : Outport  Port=3
  alpha_d : Outport  Port=4
  wires:
  [theta_d] -> Product2/3
  Gain7/1 -> Sum3/2
  [theta_d] -> Math Function1/1
  Gain3/1 -> Sum2/1
  Gain/1 -> Sum/1
  Gain2/1 -> Sum/3
  Sum3/1 -> Sum/4  "input torque"
  Fcn2/1 -> Product2/1
  [alpha] -> Fcn/1
  [alpha_dd] -> Product1/2
  [alpha_d] -> Product2/4
  [alpha] -> Fcn1/1, Fcn2/1, Fcn3/1, Fcn4/1
  Product2/1 -> Gain1/1
  Constant1/1 -> Product4/2
  [alpha] -> Fcn5/1, Fcn6/1, Fcn7/1, Fcn8/1
  Constant/1 -> Sum1/1
  Input_Voltage/1 -> Gain6/1
  Gain4/1 -> Sum2/2
  Product/1 -> Sum4/1  "theta_dd"
  Math Function/1 -> Product3/2
  Math Function1/1 -> Product6/3
  Sum2/1 -> Product4/1
  Product6/1 -> Gain4/1
  Fcn5/1 -> Product5/1
  Integrator3/1 -> alpha/1, [alpha]  "alpha"
  Product5/1 -> Gain3/1
  [theta_d] -> Gain7/1
  [theta_dd] -> Product5/2
  [alpha_d] -> Math Function/1
  Sum/1 -> Product/2
  Product3/1 -> Gain2/1
  Fcn9/1 -> Product/1
  Product1/1 -> Gain/1
  Fcn/1 -> Sum1/2
  Sum1/1 -> Fcn9/1
  Gain5/1 -> Sum2/3
  Fcn7/1 -> Product6/2
  Fcn8/1 -> Gain5/1
  Fcn1/1 -> Product1/1
  Fcn3/1 -> Product2/2
  Gain6/1 -> Sum3/1
  Gain1/1 -> Sum/2
  Integrator/1 -> Integrator1/1, [theta_d], theta_d/1  "theta_d"
  Fcn4/1 -> Product3/1
  Product4/1 -> Integrator2/1, [alpha_dd]  "alpha_dd"
  Fcn6/1 -> Product6/1
  Integrator2/1 -> [alpha_d], Integrator3/1, alpha_d/1  "alpha_d"
  [alpha_d] -> Gain8/1
  Gain8/1 -> Sum2/4
  Integrator1/1 -> theta/1, Goto5/1, Sum4/2  "theta"
  Dead Zone/1 -> Gain9/1
  [theta_d] -> Fcn10/1
  Fcn10/1 -> Sum/5
  Gain9/1 -> Sum/6
  From12/1 -> Dead Zone/1
  Sum4/1 -> [theta_dd], Integrator/1

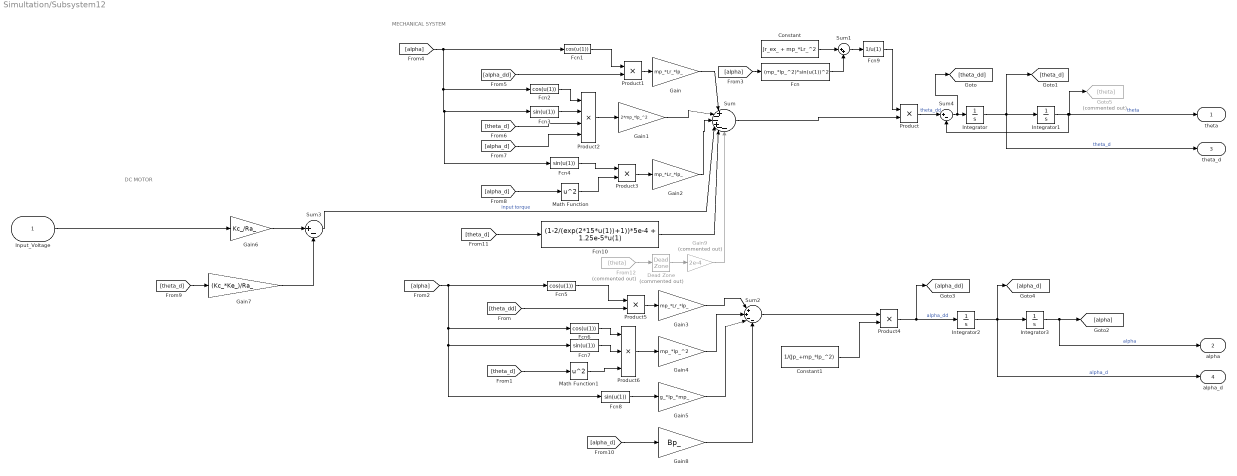
== system Simultation/Subsystem12 ==
  note: MECHANICAL SYSTEM
  note: DC MOTOR
  Input_Voltage : Inport
  Constant : Constant  Value=Jr_ex_ + mp_*Lr_^2
  Constant1 : Constant  Value=1/(Jp_+mp_*lp_^2)
  Dead Zone : DeadZone  Commented=on  LowerValue=0  UpperValue=0  ZeroCross=off
  Fcn : Fcn  Expr=(mp_*lp_^2)*sin(u(1))^2
  Fcn{1..2,5..6} (4 alike) : Fcn  Expr=cos(u(1))
  Fcn10 : Fcn  Expr=(1-2/(exp(2*15*u(1))+1))*5e-4 + 1.25e-5*u(1)
  Fcn{3..4,7..8} (4 alike) : Fcn  Expr=sin(u(1))
  Fcn9 : Fcn  Expr=1/u(1)
  From12 : From  Commented=on  GotoTag=theta
  Gain : Gain  Gain=mp_*Lr_*lp_
  Gain1 : Gain  Gain=2*mp_*lp_^2
  Gain2 : Gain  Gain=mp_*Lr_*lp_
  Gain3 : Gain  Gain=mp_*Lr_*lp_
  Gain4 : Gain  Gain=mp_*lp_^2
  Gain5 : Gain  Gain=g_*lp_*mp_
  Gain6 : Gain  Gain=Kc_/Ra_
  Gain7 : Gain  Gain=(Kc_*Ke_)/Ra_
  Gain8 : Gain  Gain=Bp_
  Gain9 : Gain  Commented=on  Gain=2e-4
  Goto5 : Goto  Commented=on  GotoTag=theta
  Integrator : Integrator
  Integrator1 : Integrator
  Integrator2 : Integrator
  Integrator3 : Integrator  InitialCondition=pi
  Math Function : Math  Operator=square
  Math Function1 : Math  Operator=square
  Product{,1,3..5} (5 alike) : Product
  Product2 : Product  Inputs=4
  Product6 : Product  Inputs=3
  Sum : Sum  Inputs=|+--+--
  Sum1 : Sum  Inputs=|++
  Sum2 : Sum  Inputs=|++--
  Sum3 : Sum  Inputs=|+-
  Sum4 : Sum  Inputs=|+-
  theta : Outport
  alpha : Outport  Port=2
  theta_d : Outport  Port=3
  alpha_d : Outport  Port=4
  wires:
  [theta_d] -> Product2/3
  Gain7/1 -> Sum3/2
  [theta_d] -> Math Function1/1
  Gain3/1 -> Sum2/1
  Gain/1 -> Sum/1
  Gain2/1 -> Sum/3
  Sum3/1 -> Sum/4  "input torque"
  Fcn2/1 -> Product2/1
  [alpha] -> Fcn/1
  [alpha_dd] -> Product1/2
  [alpha_d] -> Product2/4
  [alpha] -> Fcn1/1, Fcn2/1, Fcn3/1, Fcn4/1
  Product2/1 -> Gain1/1
  Constant1/1 -> Product4/2
  [alpha] -> Fcn5/1, Fcn6/1, Fcn7/1, Fcn8/1
  Constant/1 -> Sum1/1
  Input_Voltage/1 -> Gain6/1
  Gain4/1 -> Sum2/2
  Product/1 -> Sum4/1  "theta_dd"
  Math Function/1 -> Product3/2
  Math Function1/1 -> Product6/3
  Sum2/1 -> Product4/1
  Product6/1 -> Gain4/1
  Fcn5/1 -> Product5/1
  Integrator3/1 -> alpha/1, [alpha]  "alpha"
  Product5/1 -> Gain3/1
  [theta_d] -> Gain7/1
  [theta_dd] -> Product5/2
  [alpha_d] -> Math Function/1
  Sum/1 -> Product/2
  Product3/1 -> Gain2/1
  Fcn9/1 -> Product/1
  Product1/1 -> Gain/1
  Fcn/1 -> Sum1/2
  Sum1/1 -> Fcn9/1
  Gain5/1 -> Sum2/3
  Fcn7/1 -> Product6/2
  Fcn8/1 -> Gain5/1
  Fcn1/1 -> Product1/1
  Fcn3/1 -> Product2/2
  Gain6/1 -> Sum3/1
  Gain1/1 -> Sum/2
  Integrator/1 -> Integrator1/1, [theta_d], theta_d/1  "theta_d"
  Fcn4/1 -> Product3/1
  Product4/1 -> Integrator2/1, [alpha_dd]  "alpha_dd"
  Fcn6/1 -> Product6/1
  Integrator2/1 -> [alpha_d], Integrator3/1, alpha_d/1  "alpha_d"
  [alpha_d] -> Gain8/1
  Gain8/1 -> Sum2/4
  Integrator1/1 -> theta/1, Goto5/1, Sum4/2  "theta"
  Dead Zone/1 -> Gain9/1
  [theta_d] -> Fcn10/1
  Fcn10/1 -> Sum/5
  Gain9/1 -> Sum/6
  From12/1 -> Dead Zone/1
  Sum4/1 -> [theta_dd], Integrator/1

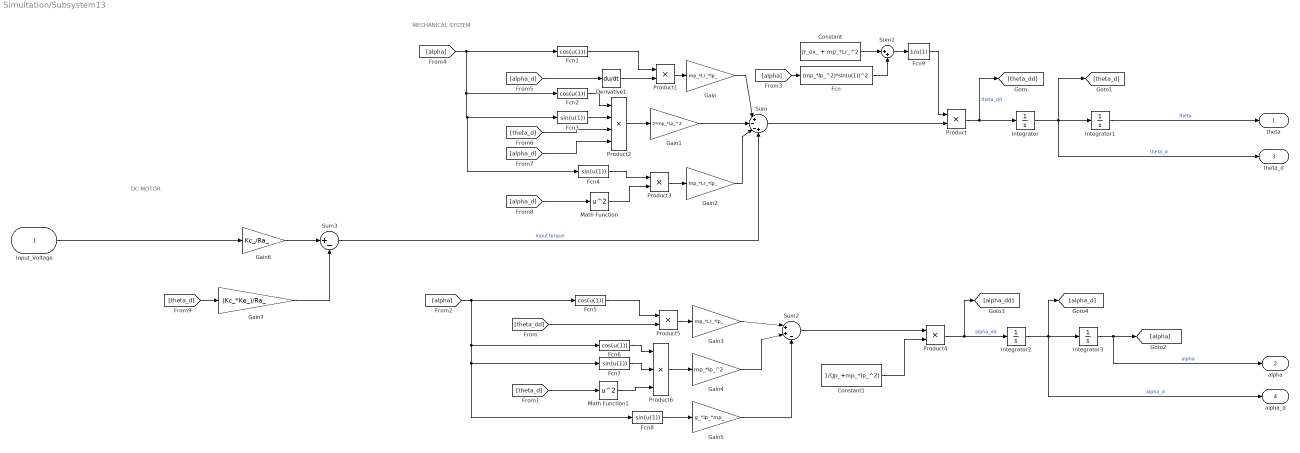
== system Simultation/Subsystem13 ==
  note: DC MOTOR
  note: MECHANICAL SYSTEM
  Input_Voltage : Inport
  Constant : Constant  Value=Jr_ex_ + mp_*Lr_^2
  Constant1 : Constant  Value=1/(Jp_+mp_*lp_^2)
  Derivative1 : Derivative
  Fcn : Fcn  Expr=(mp_*lp_^2)*sin(u(1))^2
  Fcn{1..2,5..6} (4 alike) : Fcn  Expr=cos(u(1))
  Fcn{3..4,7..8} (4 alike) : Fcn  Expr=sin(u(1))
  Fcn9 : Fcn  Expr=1/u(1)
  Gain : Gain  Gain=mp_*Lr_*lp_
  Gain1 : Gain  Gain=2*mp_*lp_^2
  Gain2 : Gain  Gain=mp_*Lr_*lp_
  Gain3 : Gain  Gain=mp_*Lr_*lp_
  Gain4 : Gain  Gain=mp_*lp_^2
  Gain5 : Gain  Gain=g_*lp_*mp_
  Gain6 : Gain  Gain=Kc_/Ra_
  Gain7 : Gain  Gain=(Kc_*Ke_)/Ra_
  Integrator{,1..3} (4 alike) : Integrator
  Math Function : Math  Operator=square
  Math Function1 : Math  Operator=square
  Product{,1,3..5} (5 alike) : Product
  Product2 : Product  Inputs=4
  Product6 : Product  Inputs=3
  Sum : Sum  Inputs=|+--+
  Sum1 : Sum  Inputs=|++
  Sum2 : Sum  Inputs=|++-
  Sum3 : Sum  Inputs=|+-
  theta : Outport
  alpha : Outport  Port=2
  theta_d : Outport  Port=3
  alpha_d : Outport  Port=4
  wires:
  Integrator2/1 -> alpha_d/1, Integrator3/1, [alpha_d]  "alpha_d"
  Fcn6/1 -> Product6/1
  Product4/1 -> [alpha_dd], Integrator2/1  "alpha_dd"
  Fcn4/1 -> Product3/1
  Integrator/1 -> theta_d/1, [theta_d], Integrator1/1  "theta_d"
  Gain6/1 -> Sum3/1
  Fcn3/1 -> Product2/2
  Fcn1/1 -> Product1/1
  Integrator1/1 -> theta/1  "theta"
  Fcn8/1 -> Gain5/1
  Fcn7/1 -> Product6/2
  Gain5/1 -> Sum2/3
  Sum1/1 -> Fcn9/1
  Fcn/1 -> Sum1/2
  Product1/1 -> Gain/1
  Fcn9/1 -> Product/1
  Product3/1 -> Gain2/1
  Sum/1 -> Product/2
  [alpha_d] -> Math Function/1
  [theta_dd] -> Product5/2
  [theta_d] -> Gain7/1
  Product5/1 -> Gain3/1
  Integrator3/1 -> alpha/1, [alpha]  "alpha"
  Fcn5/1 -> Product5/1
  Product6/1 -> Gain4/1
  Sum2/1 -> Product4/1
  Math Function1/1 -> Product6/3
  Math Function/1 -> Product3/2
  Product/1 -> Integrator/1, [theta_dd]  "theta_dd"
  Gain4/1 -> Sum2/2
  Input_Voltage/1 -> Gain6/1
  Constant/1 -> Sum1/1
  [alpha] -> Fcn8/1, Fcn7/1, Fcn6/1, Fcn5/1
  Constant1/1 -> Product4/2
  Product2/1 -> Gain1/1
  [alpha] -> Fcn4/1, Fcn3/1, Fcn2/1, Fcn1/1
  [alpha_d] -> Product2/4
  [alpha] -> Fcn/1
  Fcn2/1 -> Product2/1
  Sum3/1 -> Sum/4  "input torque"
  Gain2/1 -> Sum/3
  Gain3/1 -> Sum2/1
  [theta_d] -> Math Function1/1
  Gain7/1 -> Sum3/2
  [theta_d] -> Product2/3
  Gain1/1 -> Sum/2
  Gain/1 -> Sum/1
  [alpha_d] -> Derivative1/1
  Derivative1/1 -> Product1/2

== system Simultation/Subsystem14 ==
  note: DC MOTOR
  note: MECHANICAL SYSTEM
  Input_Voltage : Inport
  Constant : Constant  Value=Jr_ex_ + mp_*Lr_^2
  Constant1 : Constant  Value=1/(Jp_+mp_*lp_^2)
  Derivative1 : Derivative
  Fcn : Fcn  Expr=(mp_*lp_^2)*sin(u(1))^2
  Fcn{1..2,5..6} (4 alike) : Fcn  Expr=cos(u(1))
  Fcn{3..4,7..8} (4 alike) : Fcn  Expr=sin(u(1))
  Fcn9 : Fcn  Expr=1/u(1)
  Gain : Gain  Gain=mp_*Lr_*lp_
  Gain1 : Gain  Gain=2*mp_*lp_^2
  Gain2 : Gain  Gain=mp_*Lr_*lp_
  Gain3 : Gain  Gain=mp_*Lr_*lp_
  Gain4 : Gain  Gain=mp_*lp_^2
  Gain5 : Gain  Gain=g_*lp_*mp_
  Gain6 : Gain  Gain=Kc_/Ra_
  Gain7 : Gain  Gain=(Kc_*Ke_)/Ra_
  Integrator{,1..3} (4 alike) : Integrator
  Math Function : Math  Operator=square
  Math Function1 : Math  Operator=square
  Product{,1,3..5} (5 alike) : Product
  Product2 : Product  Inputs=4
  Product6 : Product  Inputs=3
  Sum : Sum  Inputs=|+--+
  Sum1 : Sum  Inputs=|++
  Sum2 : Sum  Inputs=|++-
  Sum3 : Sum  Inputs=|+-
  theta : Outport
  alpha : Outport  Port=2
  theta_d : Outport  Port=3
  alpha_d : Outport  Port=4
  wires:
  Integrator2/1 -> alpha_d/1, Integrator3/1, [alpha_d]  "alpha_d"
  Fcn6/1 -> Product6/1
  Product4/1 -> Integrator2/1  "alpha_dd"
  Fcn4/1 -> Product3/1
  Integrator/1 -> theta_d/1, [theta_d], Integrator1/1  "theta_d"
  Gain6/1 -> Sum3/1
  Fcn3/1 -> Product2/2
  Fcn1/1 -> Product1/1
  Integrator1/1 -> theta/1  "theta"
  Fcn8/1 -> Gain5/1
  Fcn7/1 -> Product6/2
  Gain5/1 -> Sum2/3
  Sum1/1 -> Fcn9/1
  Fcn/1 -> Sum1/2
  Product1/1 -> Gain/1
  Fcn9/1 -> Product/1
  Product3/1 -> Gain2/1
  Sum/1 -> Product/2
  [alpha_d] -> Math Function/1
  [theta_dd] -> Product5/2
  [theta_d] -> Gain7/1
  Product5/1 -> Gain3/1
  Integrator3/1 -> alpha/1, [alpha]  "alpha"
  Fcn5/1 -> Product5/1
  Product6/1 -> Gain4/1
  Sum2/1 -> Product4/1
  Math Function1/1 -> Product6/3
  Math Function/1 -> Product3/2
  Product/1 -> Integrator/1, [theta_dd]  "theta_dd"
  Gain4/1 -> Sum2/2
  Input_Voltage/1 -> Gain6/1
  Constant/1 -> Sum1/1
  [alpha] -> Fcn8/1, Fcn7/1, Fcn6/1, Fcn5/1
  Constant1/1 -> Product4/2
  Product2/1 -> Gain1/1
  [alpha] -> Fcn4/1, Fcn3/1, Fcn2/1, Fcn1/1
  [alpha_d] -> Product2/4
  [alpha] -> Fcn/1
  Fcn2/1 -> Product2/1
  Sum3/1 -> Sum/4  "input torque"
  Gain2/1 -> Sum/3
  Gain3/1 -> Sum2/1
  [theta_d] -> Math Function1/1
  Gain7/1 -> Sum3/2
  [theta_d] -> Product2/3
  Gain1/1 -> Sum/2
  Gain/1 -> Sum/1
  [alpha_d] -> Derivative1/1
  Derivative1/1 -> Product1/2

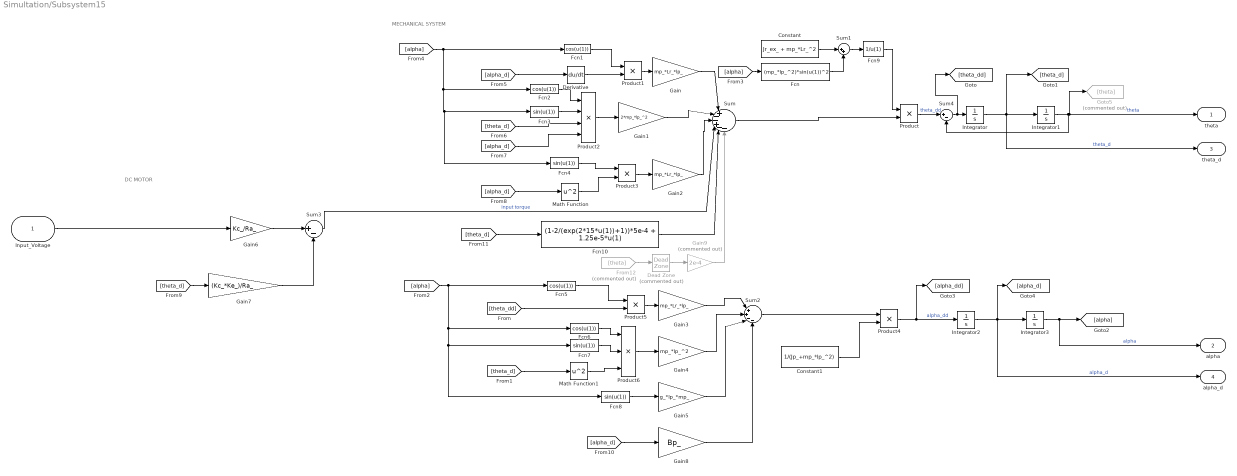
== system Simultation/Subsystem15 ==
  note: MECHANICAL SYSTEM
  note: DC MOTOR
  Input_Voltage : Inport
  Constant : Constant  Value=Jr_ex_ + mp_*Lr_^2
  Constant1 : Constant  Value=1/(Jp_+mp_*lp_^2)
  Dead Zone : DeadZone  Commented=on  LowerValue=0  UpperValue=0  ZeroCross=off
  Derivative : Derivative
  Fcn : Fcn  Expr=(mp_*lp_^2)*sin(u(1))^2
  Fcn{1..2,5..6} (4 alike) : Fcn  Expr=cos(u(1))
  Fcn10 : Fcn  Expr=(1-2/(exp(2*15*u(1))+1))*5e-4 + 1.25e-5*u(1)
  Fcn{3..4,7..8} (4 alike) : Fcn  Expr=sin(u(1))
  Fcn9 : Fcn  Expr=1/u(1)
  From12 : From  Commented=on  GotoTag=theta
  Gain : Gain  Gain=mp_*Lr_*lp_
  Gain1 : Gain  Gain=2*mp_*lp_^2
  Gain2 : Gain  Gain=mp_*Lr_*lp_
  Gain3 : Gain  Gain=mp_*Lr_*lp_
  Gain4 : Gain  Gain=mp_*lp_^2
  Gain5 : Gain  Gain=g_*lp_*mp_
  Gain6 : Gain  Gain=Kc_/Ra_
  Gain7 : Gain  Gain=(Kc_*Ke_)/Ra_
  Gain8 : Gain  Gain=Bp_
  Gain9 : Gain  Commented=on  Gain=2e-4
  Goto5 : Goto  Commented=on  GotoTag=theta
  Integrator{,1..3} (4 alike) : Integrator
  Math Function : Math  Operator=square
  Math Function1 : Math  Operator=square
  Product{,1,3..5} (5 alike) : Product
  Product2 : Product  Inputs=4
  Product6 : Product  Inputs=3
  Sum : Sum  Inputs=|+--+--
  Sum1 : Sum  Inputs=|++
  Sum2 : Sum  Inputs=|++--
  Sum3 : Sum  Inputs=|+-
  Sum4 : Sum  Inputs=|+-
  theta : Outport
  alpha : Outport  Port=2
  theta_d : Outport  Port=3
  alpha_d : Outport  Port=4
  wires:
  [theta_d] -> Product2/3
  Gain7/1 -> Sum3/2
  [theta_d] -> Math Function1/1
  Gain3/1 -> Sum2/1
  Gain/1 -> Sum/1
  Gain2/1 -> Sum/3
  Sum3/1 -> Sum/4  "input torque"
  Fcn2/1 -> Product2/1
  [alpha] -> Fcn/1
  [alpha_d] -> Product2/4
  [alpha] -> Fcn1/1, Fcn2/1, Fcn3/1, Fcn4/1
  Product2/1 -> Gain1/1
  Constant1/1 -> Product4/2
  [alpha] -> Fcn5/1, Fcn6/1, Fcn7/1, Fcn8/1
  Constant/1 -> Sum1/1
  Input_Voltage/1 -> Gain6/1
  Gain4/1 -> Sum2/2
  Product/1 -> Sum4/1  "theta_dd"
  Math Function/1 -> Product3/2
  Math Function1/1 -> Product6/3
  Sum2/1 -> Product4/1
  Product6/1 -> Gain4/1
  Fcn5/1 -> Product5/1
  Integrator3/1 -> alpha/1, [alpha]  "alpha"
  Product5/1 -> Gain3/1
  [theta_d] -> Gain7/1
  [theta_dd] -> Product5/2
  [alpha_d] -> Math Function/1
  Sum/1 -> Product/2
  Product3/1 -> Gain2/1
  Fcn9/1 -> Product/1
  Product1/1 -> Gain/1
  Fcn/1 -> Sum1/2
  Sum1/1 -> Fcn9/1
  Gain5/1 -> Sum2/3
  Fcn7/1 -> Product6/2
  Fcn8/1 -> Gain5/1
  Fcn1/1 -> Product1/1
  Fcn3/1 -> Product2/2
  Gain6/1 -> Sum3/1
  Gain1/1 -> Sum/2
  Integrator/1 -> Integrator1/1, [theta_d], theta_d/1  "theta_d"
  Fcn4/1 -> Product3/1
  Product4/1 -> Integrator2/1, [alpha_dd]  "alpha_dd"
  Fcn6/1 -> Product6/1
  Integrator2/1 -> [alpha_d], Integrator3/1, alpha_d/1  "alpha_d"
  [alpha_d] -> Gain8/1
  Gain8/1 -> Sum2/4
  Integrator1/1 -> theta/1, Goto5/1, Sum4/2  "theta"
  Dead Zone/1 -> Gain9/1
  [theta_d] -> Fcn10/1
  Fcn10/1 -> Sum/5
  Gain9/1 -> Sum/6
  From12/1 -> Dead Zone/1
  Sum4/1 -> [theta_dd], Integrator/1
  Derivative/1 -> Product1/2
  [alpha_d] -> Derivative/1

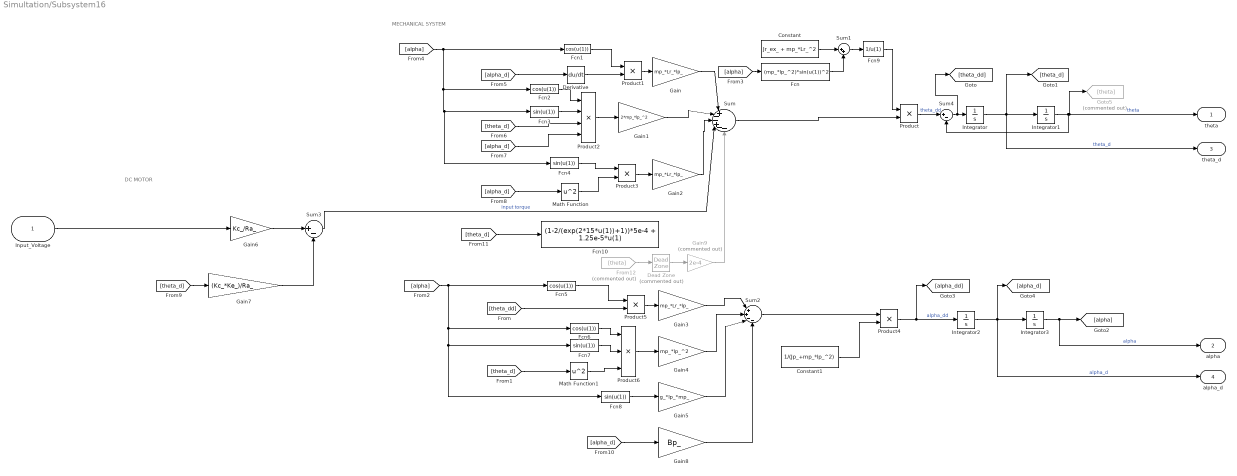
== system Simultation/Subsystem16 ==
  note: MECHANICAL SYSTEM
  note: DC MOTOR
  Input_Voltage : Inport
  Constant : Constant  Value=Jr_ex_ + mp_*Lr_^2
  Constant1 : Constant  Value=1/(Jp_+mp_*lp_^2)
  Dead Zone : DeadZone  Commented=on  LowerValue=0  UpperValue=0  ZeroCross=off
  Derivative : Derivative
  Fcn : Fcn  Expr=(mp_*lp_^2)*sin(u(1))^2
  Fcn{1..2,5..6} (4 alike) : Fcn  Expr=cos(u(1))
  Fcn10 : Fcn  Expr=(1-2/(exp(2*15*u(1))+1))*5e-4 + 1.25e-5*u(1)
  Fcn{3..4,7..8} (4 alike) : Fcn  Expr=sin(u(1))
  Fcn9 : Fcn  Expr=1/u(1)
  From12 : From  Commented=on  GotoTag=theta
  Gain : Gain  Gain=mp_*Lr_*lp_
  Gain1 : Gain  Gain=2*mp_*lp_^2
  Gain2 : Gain  Gain=mp_*Lr_*lp_
  Gain3 : Gain  Gain=mp_*Lr_*lp_
  Gain4 : Gain  Gain=mp_*lp_^2
  Gain5 : Gain  Gain=g_*lp_*mp_
  Gain6 : Gain  Gain=Kc_/Ra_
  Gain7 : Gain  Gain=(Kc_*Ke_)/Ra_
  Gain8 : Gain  Gain=Bp_
  Gain9 : Gain  Commented=on  Gain=2e-4
  Goto5 : Goto  Commented=on  GotoTag=theta
  Integrator{,1..3} (4 alike) : Integrator
  Math Function : Math  Operator=square
  Math Function1 : Math  Operator=square
  Product{,1,3..5} (5 alike) : Product
  Product2 : Product  Inputs=4
  Product6 : Product  Inputs=3
  Sum : Sum  Inputs=|+--+--
  Sum1 : Sum  Inputs=|++
  Sum2 : Sum  Inputs=|++--
  Sum3 : Sum  Inputs=|+-
  Sum4 : Sum  Inputs=|+-
  theta : Outport
  alpha : Outport  Port=2
  theta_d : Outport  Port=3
  alpha_d : Outport  Port=4
  wires:
  [theta_d] -> Product2/3
  Gain7/1 -> Sum3/2
  [theta_d] -> Math Function1/1
  Gain3/1 -> Sum2/1
  Gain/1 -> Sum/1
  Gain2/1 -> Sum/3
  Sum3/1 -> Sum/4  "input torque"
  Fcn2/1 -> Product2/1
  [alpha] -> Fcn/1
  [alpha_d] -> Product2/4
  [alpha] -> Fcn1/1, Fcn2/1, Fcn3/1, Fcn4/1
  Product2/1 -> Gain1/1
  Constant1/1 -> Product4/2
  [alpha] -> Fcn5/1, Fcn6/1, Fcn7/1, Fcn8/1
  Constant/1 -> Sum1/1
  Input_Voltage/1 -> Gain6/1
  Gain4/1 -> Sum2/2
  Product/1 -> Sum4/1  "theta_dd"
  Math Function/1 -> Product3/2
  Math Function1/1 -> Product6/3
  Sum2/1 -> Product4/1
  Product6/1 -> Gain4/1
  Fcn5/1 -> Product5/1
  Integrator3/1 -> alpha/1, [alpha]  "alpha"
  Product5/1 -> Gain3/1
  [theta_d] -> Gain7/1
  [theta_dd] -> Product5/2
  [alpha_d] -> Math Function/1
  Sum/1 -> Product/2
  Product3/1 -> Gain2/1
  Fcn9/1 -> Product/1
  Product1/1 -> Gain/1
  Fcn/1 -> Sum1/2
  Sum1/1 -> Fcn9/1
  Gain5/1 -> Sum2/3
  Fcn7/1 -> Product6/2
  Fcn8/1 -> Gain5/1
  Fcn1/1 -> Product1/1
  Fcn3/1 -> Product2/2
  Gain6/1 -> Sum3/1
  Gain1/1 -> Sum/2
  Integrator/1 -> Integrator1/1, [theta_d], theta_d/1  "theta_d"
  Fcn4/1 -> Product3/1
  Product4/1 -> Integrator2/1, [alpha_dd]  "alpha_dd"
  Fcn6/1 -> Product6/1
  Integrator2/1 -> [alpha_d], Integrator3/1, alpha_d/1  "alpha_d"
  [alpha_d] -> Gain8/1
  Gain8/1 -> Sum2/4
  Integrator1/1 -> theta/1, Goto5/1, Sum4/2  "theta"
  Dead Zone/1 -> Gain9/1
  [theta_d] -> Fcn10/1
  Gain9/1 -> Sum/6
  From12/1 -> Dead Zone/1
  Sum4/1 -> [theta_dd], Integrator/1
  Derivative/1 -> Product1/2
  [alpha_d] -> Derivative/1

== system Simultation/Subsystem17 ==
  note: DC MOTOR
  note: MECHANICAL SYSTEM
  Input_Voltage : Inport
  Constant : Constant  Value=Jr_ex_ + mp_*Lr_^2
  Constant1 : Constant  Value=1/(Jp_+mp_*lp_^2)
  Derivative1 : Derivative
  Fcn : Fcn  Expr=(mp_*lp_^2)*sin(u(1))^2
  Fcn{1..2,5..6} (4 alike) : Fcn  Expr=cos(u(1))
  Fcn{3..4,7..8} (4 alike) : Fcn  Expr=sin(u(1))
  Fcn9 : Fcn  Expr=1/u(1)
  Gain : Gain  Gain=mp_*Lr_*lp_
  Gain1 : Gain  Gain=2*mp_*lp_^2
  Gain2 : Gain  Gain=mp_*Lr_*lp_
  Gain3 : Gain  Gain=mp_*Lr_*lp_
  Gain4 : Gain  Gain=mp_*lp_^2
  Gain5 : Gain  Gain=g_*lp_*mp_
  Gain6 : Gain  Gain=Kc_/Ra_
  Gain7 : Gain  Gain=(Kc_*Ke_)/Ra_
  Integrator{,1..3} (4 alike) : Integrator
  Math Function : Math  Operator=square
  Math Function1 : Math  Operator=square
  Product{,1,3..5} (5 alike) : Product
  Product2 : Product  Inputs=4
  Product6 : Product  Inputs=3
  Sum : Sum  Inputs=|+--+
  Sum1 : Sum  Inputs=|++
  Sum2 : Sum  Inputs=|++-
  Sum3 : Sum  Inputs=|+-
  theta : Outport
  alpha : Outport  Port=2
  theta_d : Outport  Port=3
  alpha_d : Outport  Port=4
  wires:
  Integrator2/1 -> alpha_d/1, Integrator3/1, [alpha_d]  "alpha_d"
  Fcn6/1 -> Product6/1
  Product4/1 -> Integrator2/1  "alpha_dd"
  Fcn4/1 -> Product3/1
  Integrator/1 -> theta_d/1, [theta_d], Integrator1/1  "theta_d"
  Gain6/1 -> Sum3/1
  Fcn3/1 -> Product2/2
  Fcn1/1 -> Product1/1
  Integrator1/1 -> theta/1  "theta"
  Fcn8/1 -> Gain5/1
  Fcn7/1 -> Product6/2
  Gain5/1 -> Sum2/3
  Sum1/1 -> Fcn9/1
  Fcn/1 -> Sum1/2
  Product1/1 -> Gain/1
  Fcn9/1 -> Product/1
  Product3/1 -> Gain2/1
  Sum/1 -> Product/2
  [alpha_d] -> Math Function/1
  [theta_dd] -> Product5/2
  [theta_d] -> Gain7/1
  Product5/1 -> Gain3/1
  Integrator3/1 -> alpha/1, [alpha]  "alpha"
  Fcn5/1 -> Product5/1
  Product6/1 -> Gain4/1
  Sum2/1 -> Product4/1
  Math Function1/1 -> Product6/3
  Math Function/1 -> Product3/2
  Product/1 -> Integrator/1, [theta_dd]  "theta_dd"
  Gain4/1 -> Sum2/2
  Input_Voltage/1 -> Gain6/1
  Constant/1 -> Sum1/1
  [alpha] -> Fcn8/1, Fcn7/1, Fcn6/1, Fcn5/1
  Constant1/1 -> Product4/2
  Product2/1 -> Gain1/1
  [alpha] -> Fcn4/1, Fcn3/1, Fcn2/1, Fcn1/1
  [alpha_d] -> Product2/4
  [alpha] -> Fcn/1
  Fcn2/1 -> Product2/1
  Sum3/1 -> Sum/4  "input torque"
  Gain2/1 -> Sum/3
  Gain3/1 -> Sum2/1
  [theta_d] -> Math Function1/1
  Gain7/1 -> Sum3/2
  [theta_d] -> Product2/3
  Gain1/1 -> Sum/2
  Gain/1 -> Sum/1
  [alpha_d] -> Derivative1/1
  Derivative1/1 -> Product1/2

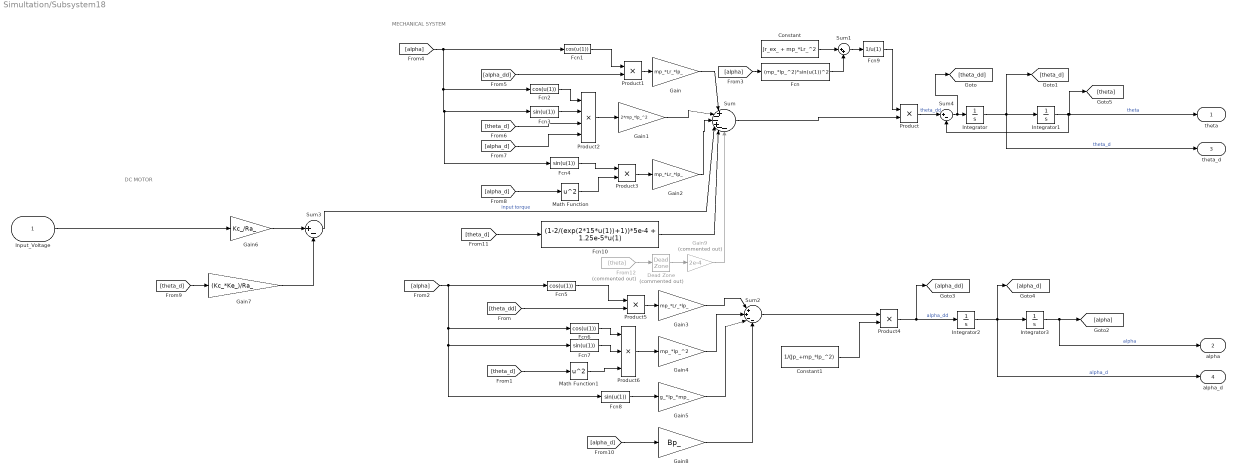
== system Simultation/Subsystem18 ==
  note: MECHANICAL SYSTEM
  note: DC MOTOR
  Input_Voltage : Inport
  Constant : Constant  Value=Jr_ex_ + mp_*Lr_^2
  Constant1 : Constant  Value=1/(Jp_+mp_*lp_^2)
  Dead Zone : DeadZone  Commented=on  LowerValue=0  UpperValue=0  ZeroCross=off
  Fcn : Fcn  Expr=(mp_*lp_^2)*sin(u(1))^2
  Fcn{1..2,5..6} (4 alike) : Fcn  Expr=cos(u(1))
  Fcn10 : Fcn  Expr=(1-2/(exp(2*15*u(1))+1))*5e-4 + 1.25e-5*u(1)
  Fcn{3..4,7..8} (4 alike) : Fcn  Expr=sin(u(1))
  Fcn9 : Fcn  Expr=1/u(1)
  From12 : From  Commented=on  GotoTag=theta
  Gain : Gain  Gain=mp_*Lr_*lp_
  Gain1 : Gain  Gain=2*mp_*lp_^2
  Gain2 : Gain  Gain=mp_*Lr_*lp_
  Gain3 : Gain  Gain=mp_*Lr_*lp_
  Gain4 : Gain  Gain=mp_*lp_^2
  Gain5 : Gain  Gain=g_*lp_*mp_
  Gain6 : Gain  Gain=Kc_/Ra_
  Gain7 : Gain  Gain=(Kc_*Ke_)/Ra_
  Gain8 : Gain  Gain=Bp_
  Gain9 : Gain  Commented=on  Gain=2e-4
  Integrator{,1..3} (4 alike) : Integrator
  Math Function : Math  Operator=square
  Math Function1 : Math  Operator=square
  Product{,1,3..5} (5 alike) : Product
  Product2 : Product  Inputs=4
  Product6 : Product  Inputs=3
  Sum : Sum  Inputs=|+--+--
  Sum1 : Sum  Inputs=|++
  Sum2 : Sum  Inputs=|++--
  Sum3 : Sum  Inputs=|+-
  Sum4 : Sum  Inputs=|+-
  theta : Outport
  alpha : Outport  Port=2
  theta_d : Outport  Port=3
  alpha_d : Outport  Port=4
  wires:
  [theta_d] -> Product2/3
  Gain7/1 -> Sum3/2
  [theta_d] -> Math Function1/1
  Gain3/1 -> Sum2/1
  Gain/1 -> Sum/1
  Gain2/1 -> Sum/3
  Sum3/1 -> Sum/4  "input torque"
  Fcn2/1 -> Product2/1
  [alpha] -> Fcn/1
  [alpha_d] -> Product2/4
  [alpha] -> Fcn1/1, Fcn2/1, Fcn3/1, Fcn4/1
  Product2/1 -> Gain1/1
  Constant1/1 -> Product4/2
  [alpha] -> Fcn5/1, Fcn6/1, Fcn7/1, Fcn8/1
  Constant/1 -> Sum1/1
  Input_Voltage/1 -> Gain6/1
  Gain4/1 -> Sum2/2
  Product/1 -> Sum4/1  "theta_dd"
  Math Function/1 -> Product3/2
  Math Function1/1 -> Product6/3
  Sum2/1 -> Product4/1
  Product6/1 -> Gain4/1
  Fcn5/1 -> Product5/1
  Integrator3/1 -> alpha/1, [alpha]  "alpha"
  Product5/1 -> Gain3/1
  [theta_d] -> Gain7/1
  [theta_dd] -> Product5/2
  [alpha_d] -> Math Function/1
  Sum/1 -> Product/2
  Product3/1 -> Gain2/1
  Fcn9/1 -> Product/1
  Product1/1 -> Gain/1
  Fcn/1 -> Sum1/2
  Sum1/1 -> Fcn9/1
  Gain5/1 -> Sum2/3
  Fcn7/1 -> Product6/2
  Fcn8/1 -> Gain5/1
  Fcn1/1 -> Product1/1
  Fcn3/1 -> Product2/2
  Gain6/1 -> Sum3/1
  Gain1/1 -> Sum/2
  Integrator/1 -> Integrator1/1, [theta_d], theta_d/1  "theta_d"
  Fcn4/1 -> Product3/1
  Product4/1 -> Integrator2/1, [alpha_dd]  "alpha_dd"
  Fcn6/1 -> Product6/1
  Integrator2/1 -> [alpha_d], Integrator3/1, alpha_d/1  "alpha_d"
  [alpha_d] -> Gain8/1
  Gain8/1 -> Sum2/4
  Integrator1/1 -> theta/1, [theta], Sum4/2  "theta"
  Dead Zone/1 -> Gain9/1
  [theta_d] -> Fcn10/1
  Gain9/1 -> Sum/6
  From12/1 -> Dead Zone/1
  Sum4/1 -> [theta_dd], Integrator/1
  [alpha_dd] -> Product1/2
  Fcn10/1 -> Sum/5
